simulink model "pv_control"  (R2023a)
settings: Solver=FixedStepDiscrete  StartTime=0.0  StopTime=Inf  FixedStep=Ts  RelTol=1e-3  EnableMultiTasking=on
undefined symbols (not defined in the file): dendp, denPQ, DiscIntNeverNeededParam, Down, Emax, fff, GPTRIP1SEL, GPTRIP2SEL, k, Kic, Kiv, Kpc, Kpv, L, l, m, n, numdp, numPQ, Ts, TZ1, TZ2, Up, Vdc, w
libraries: memblks x14, simulink x13, c2802xlib x12, slpidlib x9, c2837xDlib x7, spsdq0toabcLib x2, spsabctodq0Lib x2, dspswit3 x2, eeGeneralControl x1, idelinklib_common x1, spsPowerdq0InstantaneousLib x1, simulink_extras x1
(part 2 of 8)

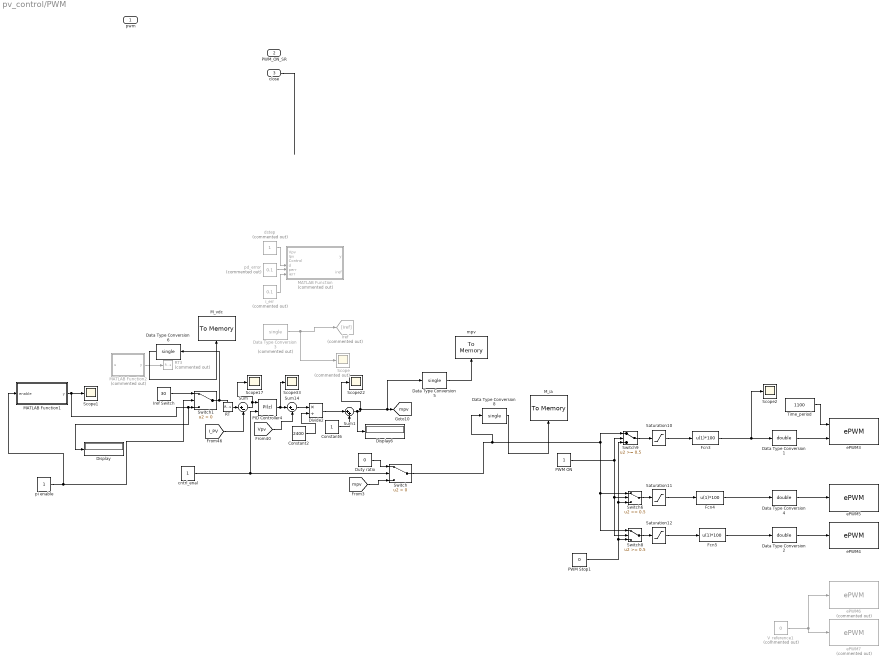
== system pv_control/PWM ==
  pwm : Inport
  PWM_ON_SR : Inport  Port=2
  close : Inport  Port=3
  Constant2 : Constant  Value=2400
  Constant6 : Constant
  Data Type Conversion1 : DataTypeConversion  OutDataTypeStr=double  SaturateOnIntegerOverflow=off  RndMeth=Floor
  Data Type Conversion2 : DataTypeConversion  OutDataTypeStr=double  SaturateOnIntegerOverflow=off  RndMeth=Floor
  Data Type Conversion3 : DataTypeConversion  Commented=on  OutDataTypeStr=single  SaturateOnIntegerOverflow=off  RndMeth=Floor
  Data Type Conversion4 : DataTypeConversion  OutDataTypeStr=double  SaturateOnIntegerOverflow=off  RndMeth=Floor
  Data Type Conversion5 : DataTypeConversion  OutDataTypeStr=single  SaturateOnIntegerOverflow=off  RndMeth=Floor
  Data Type Conversion6 : DataTypeConversion  OutDataTypeStr=single  SaturateOnIntegerOverflow=off  RndMeth=Floor
  Data Type Conversion8 : DataTypeConversion  OutDataTypeStr=single  SaturateOnIntegerOverflow=off  RndMeth=Floor
  Display : Display
  Display6 : Display
  Divide2 : Product  Inputs=*/
  Duty ratio : Constant  Value=0  OutDataTypeStr=double  SampleTime=Ts
  Fcn3 : Fcn  Expr=u(1)*100
  Fcn4 : Fcn  Expr=u(1)*100
  Fcn5 : Fcn  Expr=u(1)*100
  Iref : Goto  Commented=on  GotoTag=Iref
  Iref Switch : Constant  Value=30
  MATLAB Function : MATLAB Function  Commented=on  TreatAsAtomicUnit=on  SystemSampleTime=0.1
  MATLAB Function1 : MATLAB Function  TreatAsAtomicUnit=on  SystemSampleTime=0.0005
  MATLAB Function2 : MATLAB Function  Commented=on  TreatAsAtomicUnit=on  SystemSampleTime=0.1
  M_ia : memblks/To Memory  memAddressMask=a800  dType=single  useInitValue=off  initValue=0  useTermValue=off  termValue=0  isRealtimeEnabled=on  emitCCBeforeWrite=off  emitCCAfterWrite=on  CCAfterWrite=if(n4<200) ia[n4++]=*ia_pointer;else n4=0;
  M_vdc : memblks/To Memory  memAddressMask=a300  dType=single  useInitValue=off  initValue=0  useTermValue=off  termValue=0  isRealtimeEnabled=on  emitCCBeforeWrite=off  emitCCAfterWrite=on  CCAfterWrite=if(n7<200) vdc[n7++]=*vdc_pointer;else n7=0;
  PID Controller4 : slpidlib/PID Controller  Controller=PI  Form=Parallel  TimeDomain=Discrete-time  UseExternalTs=off  SampleTime=Ts  IntegratorMethod=Forward Euler  FilterMethod=Forward Euler  ControllerParametersSource=internal  P=1  I=40  UseKiTs=off  D=0  N=100  UseFilter=on  TunerSelectOption=Frequency Response Based  InitialConditionSource=internal  InitialConditionForIntegrator=0  InitialConditionForFilter=0  DifferentiatorICPrevScaledInput=0  ExternalReset=level  TrackingMode=off  Kt=1  LimitOutput=off  SatLimitsSource=internal  UpperSaturationLimit=inf  LowerSaturationLimit=-inf  LinearizeAsGain=on  AntiWindupMode=none  Kb=1  LimitIntegrator=off  UpperIntegratorSaturationLimit=inf  LowerIntegratorSaturationLimit=-inf  POutMin=[]  POutMax=[]  IOutMin=[]  IOutMax=[]  DOutMin=[]  DOutMax=[]  NOutMin=[]  NOutMax=[]  SumOutMin=[]  SumOutMax=[]  SaturationOutMin=[]  SaturationOutMax=[]  PParamMin=[]  PParamMax=[]  IParamMin=[]  IParamMax=[]  DParamMin=[]  DParamMax=[]  NParamMin=[]  NParamMax=[]  KbParamMin=[]  KbParamMax=[]  KtParamMin=[]  KtParamMax=[]  KbOutMin=[]  KbOutMax=[]  KtOutMin=[]  KtOutMax=[]  IntegratorOutMin=[]  IntegratorOutMax=[]  FilterOutMin=[]  FilterOutMax=[]  SumI1OutMin=[]  SumI1OutMax=[]  SumI2OutMin=[]  SumI2OutMax=[]  SumI3OutMin=[]  SumI3OutMax=[]  SumI4OutMin=[]  SumI4OutMax=[]  SumDOutMin=[]  SumDOutMax=[]  DifferentiatorOutMin=[]  DifferentiatorOutMax=[]  FilterDiffOutCoefMin=[]  FilterDiffOutCoefMax=[]  ReciprocalOutMin=[]  ReciprocalOutMax=[]  SumDenOutMin=[]  SumDenOutMax=[]  SumNumOutMin=[]  SumNumOutMax=[]  DivideOutMin=[]  DivideOutMax=[]  UdiffTsProdOutMin=[]  UdiffTsProdOutMax=[]  NTsProdOutMin=[]  NTsProdOutMax=[]  UintegralTsProdOutMin=[]  UintegralTsProdOutMax=[]  UngainTsProdOutMin=[]  UngainTsProdOutMax=[]  ClampingZeroOutDataTypeStr=Inherit: Inherit via back propagation  ClampingZeroOutMin=[]  ClampingZeroOutMax=[]  FilterDenConstantOutDataTypeStr=Inherit: Inherit via back propagation  FilterDenConstantOutMin=[]  FilterDenConstantOutMax=[]  PCopyOutDataTypeStr=Inherit: Inherit via back propagation  PCopyOutMin=[]  PCopyOutMax=[]  NCopyOutDataTypeStr=Inherit: Inherit via back propagation  NCopyOutMin=[]  NCopyOutMax=[]  IntegratorContinuousStateAttributes=''  IntegratorStateMustResolveToSignalObject=off  IntegratorRTWStateStorageClass=Auto  FilterContinuousStateAttributes=''  FilterStateMustResolveToSignalObject=off  FilterRTWStateStorageClass=Auto  ParallelPVariant=InternalParameters  IdealPVariant=Disabled  IVariant=InternalParameters  DVariant=Disabled  IntegratorVariant=Discrete  SatVariant=Disabled  AWVariant=Passthrough  PCopyVariant=Disabled  TRVariant=Disabled  FdbkBlocksVariant=Forward  IdealPFdbkVariant=Disabled  SatFdbkVariant=Disabled  DerivativeFilterVariant=Disabled  NVariant=Disabled  NCopyVariant=Disabled_SignalSpec  FilterICVariant=Disabled  IntegratorICVariant=InternalICs  ExternalResetVariant=ExternalReset  TRSumVariant=Passthrough  SumFdbkVariant=Disabled  SumVariant=Sum_PI  TsampFilterVariant=InternalTs  TsampNgainVariant=Passthrough  TsampIntegralVariant=Disabled_SignalSpec  ExternalSaturationOutDataTypeStr=Inherit: Same as second input
  PWM ON : Constant
  PWM Stop1 : Constant  Value=0  OutDataTypeStr=single  SampleTime=Ts
  RT : RateTransition  OutPortSampleTime=1e-05
  RT3 : RateTransition  Commented=on  OutPortSampleTime=Ts
  Saturation10 : Saturate  UpperLimit=1  LowerLimit=0  OutDataTypeStr=double
  Saturation11 : Saturate  UpperLimit=1  LowerLimit=0  OutDataTypeStr=double
  Saturation12 : Saturate  UpperLimit=1  LowerLimit=0  OutDataTypeStr=double
  Scope : Scope  Commented=on
  Scope{1..2,17,22,33} (5 alike) : Scope
  Sum : Sum  Inputs=|+-
  Sum1 : Sum  Inputs=|++
  Sum14 : Sum  Inputs=|+-
  Switch : Switch  Criteria=u2 > Threshold  SaturateOnIntegerOverflow=off  InputSameDT=off
  Switch1 : Switch  Criteria=u2 > Threshold  OutDataTypeStr=single  SaturateOnIntegerOverflow=off  InputSameDT=off
  Switch6 : Switch  Threshold=0.5  OutDataTypeStr=single  SaturateOnIntegerOverflow=off  InputSameDT=off
  Switch8 : Switch  Threshold=0.5  OutDataTypeStr=single  SaturateOnIntegerOverflow=off  InputSameDT=off
  Switch9 : Switch  Threshold=0.5  OutDataTypeStr=single  SaturateOnIntegerOverflow=off  InputSameDT=off
  Time_period : Constant  Value=1100  OutDataTypeStr=double  SampleTime=Ts
  V_reference1 : Constant  Commented=on  Value=0  OutDataTypeStr=double  SampleTime=Ts
  cntrl_enal : Constant
  dstep : Constant  Commented=on  OutDataTypeStr=single
  ePWM3 : c2802xlib/ePWM  PwmType=C2000_Type4  useModule=ePWM4  ePWMxLINKTBPRD=Not Linked  periodUnits=Clock cycles  timerSource=Input port  timerPeriod_clk=10000  timerPeriod_sec=0.0001  tbshadow=Counter equals to zero  countingMode=Up-Down  phaseActiveEnable=Disable  phaseDirection=Count up after sync  phaseActive=0  synchronizationEnable=off  dcaevt1Sync=off  dcbevt1Sync=off  synchronizationOption=Disable  dcbevt1SyncOut=off  dcaevt1SyncOut=off  cmpdSyncOut=off  cmpcSyncOut=off  cmpbSyncOut=off  zeroSyncOut=off  swfSyncOut=off  perSynchronizationOption=Counter equals to period (CTR=PRD)  clockPrescale=1  HSclockPrescale=1  enswap=off  ePWMxAStatus=on  ePWMxAactionLogic1=Set  ePWMxAactionLogic2=Do nothing  ePWMxAactionLogic3=Clear  ePWMxAactionLogic4=Set  ePWMxAactionLogic5=Do nothing  ePWMxAactionLogic6=Do nothing  ePWMxACSFenable=off  ePWMxACSFvalue=Forcing disable  ePWMxASFreload=Zero  ePWMxBStatus=off  ePWMxBactionLogic1=Set  ePWMxBactionLogic2=Do nothing  ePWMxBactionLogic3=Clear  ePWMxBactionLogic4=Set  ePWMxBactionLogic5=Do nothing  ePWMxBactionLogic6=Do nothing  ePWMxBCSFenable=off  ePWMxBCSFvalue=Forcing low  ePWMxBSFreload=Zero  ePWNxBOutWay=off  ePWMxLINKCMPA=Not Linked  CMPAUnits=Percentages  CMPASource=Input port  CMPAValue_per=0  CMPAValue_clk=0  enCMPAshadow=Counter equals to zero (CTR=Zero)  ePWMxLINKCMPB=Not Linked  CMPBUnits=Clock cycles  CMPBSource=Specify via dialog  CMPBValue_per=50  CMPBValue_clk=3277  enCMPBshadow=Counter equals to zero (CTR=Zero)  ePWMxLINKCMPC=Not Linked  CMPCUnits=Clock cycles  CMPCSource=Specify via dialog  CMPCValue_per=50  CMPCValue_clk=3277  enCMPCshadow=Counter equals to zero (CTR=Zero)  ePWMxLINKCMPD=Not Linked  CMPDUnits=Clock cycles  CMPDSource=Specify via dialog  CMPDValue_per=50  CMPDValue_clk=3277  enCMPDshadow=Counter equals to zero (CTR=Zero)  enableDBePWMxA=on  enableDBePWMxB=on  enhalfcycle=off  DBpolarity=Active high complementary (AHC)  DBedgeDelay=Positive  DBSource_ePWMxA=ePWMxA  DBSource_ePWMxB=ePWMxA  DBPeriodUnits=Clock cycles  DBperiodSource=Specify via dialog  REDperiod=122  FEDperiod=122  REDperiod_sec=0  FEDperiod_sec=0  LoadModeDBRED=Immediate without using shadow  LoadModeDBFED=Immediate without using shadow  adcstartModuleA=on  adcrequestEventA=First event  adcstartEventA=Digital Compare Module A Event 1 start of conversion (DCAEVT1.soc)  adcstartEventA_type2=Counter equals to zero or period (CTR=Zero or CTR=PRD)  adcstartModuleB=off  adcrequestEventB=First event  adcstartEventB=Counter equals to zero (CTR=Zero)  adcstartEventB_type2=Counter equals to zero (CTR=Zero)  intEn=off  intPrd=First event  intSel=Counter equals to zero (CTR=Zero)  intSel_type2=Counter equals to zero (CTR=Zero)  hrpe=on  enHRPWM=on  HRPWM_LoadMode=Counter equals to period (CTR=PRD)  HRPWM_CTLMode=Duty or Period control mode  HRPWM_EDGMode=Both edge  hrpeb=off  enHRPWMB=off  HRPWM_LoadModeB=Counter equals to zero (CTR=ZERO)  HRPWM_CTLModeB=Duty or Period control mode  HRPWM_EDGModeB=Both edge  enHRDBRED=off  enHRDBFED=off  enSFO=on  enautoconv=on  chopperEnable=off  chopperFrequency=1  chopperFirstwidth=1  chopperDuty=12.5%  tripZonesource=Specify via dialog  tzselOSHT1=off  tzselOSHT2=off  tzselOSHT3=off  tzselOSHDCAEV1=off  tzselOSHDCBEV1=off  tzselCBC1=off  tzselCBC2=off  tzselCBC3=off  tzselCBCDCAEV2=off  tzselCBCDCBEV2=off  tzselOSHT4=off  tzselOSHT5=off  tzselOSHT6=off  tzselCBC4=off  tzselCBC5=off  tzselCBC6=off  enTzOstIntr=off  enTzCbcIntr=off  enTzDCAEVT1Intr=off  enTzDCAEVT2Intr=off  enTzDCBEVT1Intr=off  enTzDCBEVT2Intr=off  ePWMxAforced=No action  ePWMxBforced=No action  DCAEVT1forced=No action  DCBEVT1forced=No action  DCAEVT2forced=No action  DCBEVT2forced=No action  dcah=Trip Zone 1 input (TZ1)  dcal=Trip Zone 2 input (TZ2)  dcbh=Trip Zone 1 input (TZ1)  dcbl=Trip Zone 2 input (TZ2)  dcah_type2=GPTRIP1SEL/(TZ1)  dcal_type2=GPTRIP2SEL/(TZ2)  dcbh_type2=GPTRIP1SEL/(TZ1)  dcbl_type2=GPTRIP2SEL/(TZ2)  gendcaevt1=Event disabled  gendcaevt2=Event disabled  gendcbevt1=Event disabled  gendcbevt2=Event disabled  dcaevt1src=DCAEVT1 with sync  dcaevt2src=DCAEVT2 with sync  dcbevt1src=DCBEVT1 with sync  dcbevt2src=DCBEVT2 with sync  pulsesel=Counter equals to zero (CTR=Zero)  blankinv=off  blankoffset=0  blankwidth=0  evsrcsel=Filtered version of DCAEVT1 (DCAEVT1FILT)  encape=off
  ePWM4 : c2802xlib/ePWM  PwmType=C2000_Type4  useModule=ePWM3  ePWMxLINKTBPRD=Not Linked  periodUnits=Clock cycles  timerSource=Specify via dialog  timerPeriod_clk=4687  timerPeriod_sec=0.0001  tbshadow=Counter equals to zero  countingMode=Up-Down  phaseActiveEnable=Disable  phaseDirection=Count down after sync  phaseActive=0  synchronizationEnable=off  dcaevt1Sync=off  dcbevt1Sync=off  synchronizationOption=Disable  dcbevt1SyncOut=off  dcaevt1SyncOut=off  cmpdSyncOut=off  cmpcSyncOut=off  cmpbSyncOut=off  zeroSyncOut=off  swfSyncOut=off  perSynchronizationOption=Counter equals to period (CTR=PRD)  clockPrescale=1  HSclockPrescale=1  enswap=off  ePWMxAStatus=on  ePWMxAactionLogic1=Set  ePWMxAactionLogic2=Do nothing  ePWMxAactionLogic3=Clear  ePWMxAactionLogic4=Set  ePWMxAactionLogic5=Do nothing  ePWMxAactionLogic6=Do nothing  ePWMxACSFenable=off  ePWMxACSFvalue=Forcing disable  ePWMxASFreload=Zero  ePWMxBStatus=off  ePWMxBactionLogic1=Set  ePWMxBactionLogic2=Do nothing  ePWMxBactionLogic3=Clear  ePWMxBactionLogic4=Set  ePWMxBactionLogic5=Do nothing  ePWMxBactionLogic6=Do nothing  ePWMxBCSFenable=off  ePWMxBCSFvalue=Forcing disable  ePWMxBSFreload=Zero  ePWNxBOutWay=on  ePWMxLINKCMPA=Not Linked  CMPAUnits=Percentages  CMPASource=Input port  CMPAValue_per=0  CMPAValue_clk=0  enCMPAshadow=Counter equals to zero (CTR=Zero)  ePWMxLINKCMPB=Not Linked  CMPBUnits=Clock cycles  CMPBSource=Specify via dialog  CMPBValue_per=50  CMPBValue_clk=3277  enCMPBshadow=Counter equals to zero (CTR=Zero)  ePWMxLINKCMPC=Not Linked  CMPCUnits=Clock cycles  CMPCSource=Specify via dialog  CMPCValue_per=50  CMPCValue_clk=3277  enCMPCshadow=Counter equals to zero (CTR=Zero)  ePWMxLINKCMPD=Not Linked  CMPDUnits=Clock cycles  CMPDSource=Specify via dialog  CMPDValue_per=50  CMPDValue_clk=3277  enCMPDshadow=Counter equals to zero (CTR=Zero)  enableDBePWMxA=on  enableDBePWMxB=on  enhalfcycle=off  DBpolarity=Active high complementary (AHC)  DBedgeDelay=Positive  DBSource_ePWMxA=ePWMxA  DBSource_ePWMxB=ePWMxA  DBPeriodUnits=Clock cycles  DBperiodSource=Specify via dialog  REDperiod=122  FEDperiod=122  REDperiod_sec=0  FEDperiod_sec=0  LoadModeDBRED=Immediate without using shadow  LoadModeDBFED=Immediate without using shadow  adcstartModuleA=off  adcrequestEventA=First event  adcstartEventA=Digital Compare Module A Event 1 start of conversion (DCAEVT1.soc)  adcstartEventA_type2=Counter equals to zero or period (CTR=Zero or CTR=PRD)  adcstartModuleB=off  adcrequestEventB=First event  adcstartEventB=Counter equals to zero (CTR=Zero)  adcstartEventB_type2=Counter equals to zero (CTR=Zero)  intEn=off  intPrd=First event  intSel=Counter equals to zero (CTR=Zero)  intSel_type2=Counter equals to zero (CTR=Zero)  hrpe=on  enHRPWM=on  HRPWM_LoadMode=Counter equals to period (CTR=PRD)  HRPWM_CTLMode=Duty or Period control mode  HRPWM_EDGMode=Both edge  hrpeb=off  enHRPWMB=off  HRPWM_LoadModeB=Counter equals to zero (CTR=ZERO)  HRPWM_CTLModeB=Duty or Period control mode  HRPWM_EDGModeB=Both edge  enHRDBRED=off  enHRDBFED=off  enSFO=on  enautoconv=on  chopperEnable=off  chopperFrequency=1  chopperFirstwidth=1  chopperDuty=12.5%  tripZonesource=Specify via dialog  tzselOSHT1=off  tzselOSHT2=off  tzselOSHT3=off  tzselOSHDCAEV1=off  tzselOSHDCBEV1=off  tzselCBC1=off  tzselCBC2=off  tzselCBC3=off  tzselCBCDCAEV2=off  tzselCBCDCBEV2=off  tzselOSHT4=off  tzselOSHT5=off  tzselOSHT6=off  tzselCBC4=off  tzselCBC5=off  tzselCBC6=off  enTzOstIntr=off  enTzCbcIntr=off  enTzDCAEVT1Intr=off  enTzDCAEVT2Intr=off  enTzDCBEVT1Intr=off  enTzDCBEVT2Intr=off  ePWMxAforced=No action  ePWMxBforced=No action  DCAEVT1forced=No action  DCBEVT1forced=No action  DCAEVT2forced=No action  DCBEVT2forced=No action  dcah=Trip Zone 1 input (TZ1)  dcal=Trip Zone 2 input (TZ2)  dcbh=Trip Zone 1 input (TZ1)  dcbl=Trip Zone 2 input (TZ2)  dcah_type2=GPTRIP1SEL/(TZ1)  dcal_type2=GPTRIP2SEL/(TZ2)  dcbh_type2=GPTRIP1SEL/(TZ1)  dcbl_type2=GPTRIP2SEL/(TZ2)  gendcaevt1=Event disabled  gendcaevt2=Event disabled  gendcbevt1=Event disabled  gendcbevt2=Event disabled  dcaevt1src=DCAEVT1 with sync  dcaevt2src=DCAEVT2 with sync  dcbevt1src=DCBEVT1 with sync  dcbevt2src=DCBEVT2 with sync  pulsesel=Counter equals to zero (CTR=Zero)  blankinv=off  blankoffset=0  blankwidth=0  evsrcsel=Filtered version of DCAEVT1 (DCAEVT1FILT)  encape=off
  ePWM5 : c2802xlib/ePWM  PwmType=C2000_Type4  useModule=ePWM2  ePWMxLINKTBPRD=Not Linked  periodUnits=Clock cycles  timerSource=Specify via dialog  timerPeriod_clk=4687  timerPeriod_sec=0.0001  tbshadow=Counter equals to zero  countingMode=Up-Down  phaseActiveEnable=Disable  phaseDirection=Count down after sync  phaseActive=0  synchronizationEnable=off  dcaevt1Sync=off  dcbevt1Sync=off  synchronizationOption=Disable  dcbevt1SyncOut=off  dcaevt1SyncOut=off  cmpdSyncOut=off  cmpcSyncOut=off  cmpbSyncOut=off  zeroSyncOut=off  swfSyncOut=off  perSynchronizationOption=Counter equals to period (CTR=PRD)  clockPrescale=1  HSclockPrescale=1  enswap=off  ePWMxAStatus=on  ePWMxAactionLogic1=Set  ePWMxAactionLogic2=Do nothing  ePWMxAactionLogic3=Clear  ePWMxAactionLogic4=Set  ePWMxAactionLogic5=Do nothing  ePWMxAactionLogic6=Do nothing  ePWMxACSFenable=off  ePWMxACSFvalue=Forcing disable  ePWMxASFreload=Zero  ePWMxBStatus=on  ePWMxBactionLogic1=Set  ePWMxBactionLogic2=Do nothing  ePWMxBactionLogic3=Clear  ePWMxBactionLogic4=Set  ePWMxBactionLogic5=Do nothing  ePWMxBactionLogic6=Do nothing  ePWMxBCSFenable=off  ePWMxBCSFvalue=Forcing disable  ePWMxBSFreload=Zero  ePWNxBOutWay=on  ePWMxLINKCMPA=Not Linked  CMPAUnits=Percentages  CMPASource=Input port  CMPAValue_per=0  CMPAValue_clk=0  enCMPAshadow=Counter equals to zero (CTR=Zero)  ePWMxLINKCMPB=Not Linked  CMPBUnits=Clock cycles  CMPBSource=Specify via dialog  CMPBValue_per=50  CMPBValue_clk=3277  enCMPBshadow=Counter equals to zero (CTR=Zero)  ePWMxLINKCMPC=Not Linked  CMPCUnits=Clock cycles  CMPCSource=Specify via dialog  CMPCValue_per=50  CMPCValue_clk=3277  enCMPCshadow=Counter equals to zero (CTR=Zero)  ePWMxLINKCMPD=Not Linked  CMPDUnits=Clock cycles  CMPDSource=Specify via dialog  CMPDValue_per=50  CMPDValue_clk=3277  enCMPDshadow=Counter equals to zero (CTR=Zero)  enableDBePWMxA=on  enableDBePWMxB=on  enhalfcycle=off  DBpolarity=Active high complementary (AHC)  DBedgeDelay=Positive  DBSource_ePWMxA=ePWMxA  DBSource_ePWMxB=ePWMxA  DBPeriodUnits=Clock cycles  DBperiodSource=Specify via dialog  REDperiod=122  FEDperiod=122  REDperiod_sec=0  FEDperiod_sec=0  LoadModeDBRED=Immediate without using shadow  LoadModeDBFED=Immediate without using shadow  adcstartModuleA=on  adcrequestEventA=First event  adcstartEventA=Digital Compare Module A Event 1 start of conversion (DCAEVT1.soc)  adcstartEventA_type2=Counter equals to zero or period (CTR=Zero or CTR=PRD)  adcstartModuleB=off  adcrequestEventB=First event  adcstartEventB=Counter equals to zero (CTR=Zero)  adcstartEventB_type2=Counter equals to zero (CTR=Zero)  intEn=off  intPrd=First event  intSel=Counter equals to zero (CTR=Zero)  intSel_type2=Counter equals to zero (CTR=Zero)  hrpe=on  enHRPWM=on  HRPWM_LoadMode=Counter equals to period (CTR=PRD)  HRPWM_CTLMode=Duty or Period control mode  HRPWM_EDGMode=Both edge  hrpeb=off  enHRPWMB=off  HRPWM_LoadModeB=Counter equals to zero (CTR=ZERO)  HRPWM_CTLModeB=Duty or Period control mode  HRPWM_EDGModeB=Both edge  enHRDBRED=off  enHRDBFED=off  enSFO=on  enautoconv=on  chopperEnable=off  chopperFrequency=1  chopperFirstwidth=1  chopperDuty=12.5%  tripZonesource=Specify via dialog  tzselOSHT1=off  tzselOSHT2=off  tzselOSHT3=off  tzselOSHDCAEV1=off  tzselOSHDCBEV1=off  tzselCBC1=off  tzselCBC2=off  tzselCBC3=off  tzselCBCDCAEV2=off  tzselCBCDCBEV2=off  tzselOSHT4=off  tzselOSHT5=off  tzselOSHT6=off  tzselCBC4=off  tzselCBC5=off  tzselCBC6=off  enTzOstIntr=off  enTzCbcIntr=off  enTzDCAEVT1Intr=off  enTzDCAEVT2Intr=off  enTzDCBEVT1Intr=off  enTzDCBEVT2Intr=off  ePWMxAforced=No action  ePWMxBforced=No action  DCAEVT1forced=No action  DCBEVT1forced=No action  DCAEVT2forced=No action  DCBEVT2forced=No action  dcah=Trip Zone 1 input (TZ1)  dcal=Trip Zone 2 input (TZ2)  dcbh=Trip Zone 1 input (TZ1)  dcbl=Trip Zone 2 input (TZ2)  dcah_type2=GPTRIP1SEL/(TZ1)  dcal_type2=GPTRIP2SEL/(TZ2)  dcbh_type2=GPTRIP1SEL/(TZ1)  dcbl_type2=GPTRIP2SEL/(TZ2)  gendcaevt1=Event disabled  gendcaevt2=Event disabled  gendcbevt1=Event disabled  gendcbevt2=Event disabled  dcaevt1src=DCAEVT1 with sync  dcaevt2src=DCAEVT2 with sync  dcbevt1src=DCBEVT1 with sync  dcbevt2src=DCBEVT2 with sync  pulsesel=Counter equals to zero (CTR=Zero)  blankinv=off  blankoffset=0  blankwidth=0  evsrcsel=Filtered version of DCAEVT1 (DCAEVT1FILT)  encape=off
  ePWM6 : c2802xlib/ePWM  Commented=on  PwmType=C2000_Type4  useModule=ePWM5  ePWMxLINKTBPRD=Not Linked  periodUnits=Clock cycles  timerSource=Specify via dialog  timerPeriod_clk=4687  timerPeriod_sec=0.0001  tbshadow=Counter equals to zero  countingMode=Up-Down  phaseActiveEnable=Disable  phaseDirection=Count down after sync  phaseActive=0  synchronizationEnable=off  dcaevt1Sync=off  dcbevt1Sync=off  synchronizationOption=Disable  dcbevt1SyncOut=off  dcaevt1SyncOut=off  cmpdSyncOut=off  cmpcSyncOut=off  cmpbSyncOut=off  zeroSyncOut=off  swfSyncOut=off  perSynchronizationOption=Counter equals to period (CTR=PRD)  clockPrescale=1  HSclockPrescale=1  enswap=off  ePWMxAStatus=on  ePWMxAactionLogic1=Set  ePWMxAactionLogic2=Do nothing  ePWMxAactionLogic3=Clear  ePWMxAactionLogic4=Set  ePWMxAactionLogic5=Do nothing  ePWMxAactionLogic6=Do nothing  ePWMxACSFenable=off  ePWMxACSFvalue=Forcing disable  ePWMxASFreload=Zero  ePWMxBStatus=off  ePWMxBactionLogic1=Set  ePWMxBactionLogic2=Do nothing  ePWMxBactionLogic3=Clear  ePWMxBactionLogic4=Set  ePWMxBactionLogic5=Do nothing  ePWMxBactionLogic6=Do nothing  ePWMxBCSFenable=off  ePWMxBCSFvalue=Forcing disable  ePWMxBSFreload=Zero  ePWNxBOutWay=off  ePWMxLINKCMPA=Not Linked  CMPAUnits=Percentages  CMPASource=Input port  CMPAValue_per=0  CMPAValue_clk=0  enCMPAshadow=Counter equals to zero (CTR=Zero)  ePWMxLINKCMPB=Not Linked  CMPBUnits=Clock cycles  CMPBSource=Specify via dialog  CMPBValue_per=50  CMPBValue_clk=3277  enCMPBshadow=Counter equals to zero (CTR=Zero)  ePWMxLINKCMPC=Not Linked  CMPCUnits=Clock cycles  CMPCSource=Specify via dialog  CMPCValue_per=50  CMPCValue_clk=3277  enCMPCshadow=Counter equals to zero (CTR=Zero)  ePWMxLINKCMPD=Not Linked  CMPDUnits=Clock cycles  CMPDSource=Specify via dialog  CMPDValue_per=50  CMPDValue_clk=3277  enCMPDshadow=Counter equals to zero (CTR=Zero)  enableDBePWMxA=on  enableDBePWMxB=on  enhalfcycle=off  DBpolarity=Active high complementary (AHC)  DBedgeDelay=Positive  DBSource_ePWMxA=ePWMxA  DBSource_ePWMxB=ePWMxA  DBPeriodUnits=Clock cycles  DBperiodSource=Specify via dialog  REDperiod=122  FEDperiod=122  REDperiod_sec=0  FEDperiod_sec=0  LoadModeDBRED=Immediate without using shadow  LoadModeDBFED=Immediate without using shadow  adcstartModuleA=on  adcrequestEventA=First event  adcstartEventA=Digital Compare Module A Event 1 start of conversion (DCAEVT1.soc)  adcstartEventA_type2=Counter equals to zero or period (CTR=Zero or CTR=PRD)  adcstartModuleB=off  adcrequestEventB=First event  adcstartEventB=Counter equals to zero (CTR=Zero)  adcstartEventB_type2=Counter equals to zero (CTR=Zero)  intEn=off  intPrd=First event  intSel=Counter equals to zero (CTR=Zero)  intSel_type2=Counter equals to zero (CTR=Zero)  hrpe=on  enHRPWM=on  HRPWM_LoadMode=Counter equals to period (CTR=PRD)  HRPWM_CTLMode=Duty or Period control mode  HRPWM_EDGMode=Both edge  hrpeb=off  enHRPWMB=off  HRPWM_LoadModeB=Counter equals to zero (CTR=ZERO)  HRPWM_CTLModeB=Duty or Period control mode  HRPWM_EDGModeB=Both edge  enHRDBRED=off  enHRDBFED=off  enSFO=on  enautoconv=on  chopperEnable=off  chopperFrequency=1  chopperFirstwidth=1  chopperDuty=12.5%  tripZonesource=Specify via dialog  tzselOSHT1=off  tzselOSHT2=off  tzselOSHT3=off  tzselOSHDCAEV1=off  tzselOSHDCBEV1=off  tzselCBC1=off  tzselCBC2=off  tzselCBC3=off  tzselCBCDCAEV2=off  tzselCBCDCBEV2=off  tzselOSHT4=off  tzselOSHT5=off  tzselOSHT6=off  tzselCBC4=off  tzselCBC5=off  tzselCBC6=off  enTzOstIntr=off  enTzCbcIntr=off  enTzDCAEVT1Intr=off  enTzDCAEVT2Intr=off  enTzDCBEVT1Intr=off  enTzDCBEVT2Intr=off  ePWMxAforced=No action  ePWMxBforced=No action  DCAEVT1forced=No action  DCBEVT1forced=No action  DCAEVT2forced=No action  DCBEVT2forced=No action  dcah=Trip Zone 1 input (TZ1)  dcal=Trip Zone 2 input (TZ2)  dcbh=Trip Zone 1 input (TZ1)  dcbl=Trip Zone 2 input (TZ2)  dcah_type2=GPTRIP1SEL/(TZ1)  dcal_type2=GPTRIP2SEL/(TZ2)  dcbh_type2=GPTRIP1SEL/(TZ1)  dcbl_type2=GPTRIP2SEL/(TZ2)  gendcaevt1=Event disabled  gendcaevt2=Event disabled  gendcbevt1=Event disabled  gendcbevt2=Event disabled  dcaevt1src=DCAEVT1 with sync  dcaevt2src=DCAEVT2 with sync  dcbevt1src=DCBEVT1 with sync  dcbevt2src=DCBEVT2 with sync  pulsesel=Counter equals to zero (CTR=Zero)  blankinv=off  blankoffset=0  blankwidth=0  evsrcsel=Filtered version of DCAEVT1 (DCAEVT1FILT)  encape=off
  ePWM7 : c2802xlib/ePWM  Commented=on  PwmType=C2000_Type4  useModule=ePWM6  ePWMxLINKTBPRD=Not Linked  periodUnits=Clock cycles  timerSource=Specify via dialog  timerPeriod_clk=4687  timerPeriod_sec=0.0001  tbshadow=Counter equals to zero  countingMode=Up-Down  phaseActiveEnable=Disable  phaseDirection=Count down after sync  phaseActive=0  synchronizationEnable=off  dcaevt1Sync=off  dcbevt1Sync=off  synchronizationOption=Disable  dcbevt1SyncOut=off  dcaevt1SyncOut=off  cmpdSyncOut=off  cmpcSyncOut=off  cmpbSyncOut=off  zeroSyncOut=off  swfSyncOut=off  perSynchronizationOption=Counter equals to period (CTR=PRD)  clockPrescale=1  HSclockPrescale=1  enswap=off  ePWMxAStatus=on  ePWMxAactionLogic1=Set  ePWMxAactionLogic2=Do nothing  ePWMxAactionLogic3=Clear  ePWMxAactionLogic4=Set  ePWMxAactionLogic5=Do nothing  ePWMxAactionLogic6=Do nothing  ePWMxACSFenable=off  ePWMxACSFvalue=Forcing disable  ePWMxASFreload=Zero  ePWMxBStatus=off  ePWMxBactionLogic1=Set  ePWMxBactionLogic2=Do nothing  ePWMxBactionLogic3=Clear  ePWMxBactionLogic4=Set  ePWMxBactionLogic5=Do nothing  ePWMxBactionLogic6=Do nothing  ePWMxBCSFenable=off  ePWMxBCSFvalue=Forcing disable  ePWMxBSFreload=Zero  ePWNxBOutWay=off  ePWMxLINKCMPA=Not Linked  CMPAUnits=Percentages  CMPASource=Input port  CMPAValue_per=0  CMPAValue_clk=0  enCMPAshadow=Counter equals to zero (CTR=Zero)  ePWMxLINKCMPB=Not Linked  CMPBUnits=Clock cycles  CMPBSource=Specify via dialog  CMPBValue_per=50  CMPBValue_clk=3277  enCMPBshadow=Counter equals to zero (CTR=Zero)  ePWMxLINKCMPC=Not Linked  CMPCUnits=Clock cycles  CMPCSource=Specify via dialog  CMPCValue_per=50  CMPCValue_clk=3277  enCMPCshadow=Counter equals to zero (CTR=Zero)  ePWMxLINKCMPD=Not Linked  CMPDUnits=Clock cycles  CMPDSource=Specify via dialog  CMPDValue_per=50  CMPDValue_clk=3277  enCMPDshadow=Counter equals to zero (CTR=Zero)  enableDBePWMxA=on  enableDBePWMxB=on  enhalfcycle=off  DBpolarity=Active high complementary (AHC)  DBedgeDelay=Positive  DBSource_ePWMxA=ePWMxA  DBSource_ePWMxB=ePWMxA  DBPeriodUnits=Clock cycles  DBperiodSource=Specify via dialog  REDperiod=122  FEDperiod=122  REDperiod_sec=0  FEDperiod_sec=0  LoadModeDBRED=Immediate without using shadow  LoadModeDBFED=Immediate without using shadow  adcstartModuleA=on  adcrequestEventA=First event  adcstartEventA=Digital Compare Module A Event 1 start of conversion (DCAEVT1.soc)  adcstartEventA_type2=Counter equals to zero or period (CTR=Zero or CTR=PRD)  adcstartModuleB=off  adcrequestEventB=First event  adcstartEventB=Counter equals to zero (CTR=Zero)  adcstartEventB_type2=Counter equals to zero (CTR=Zero)  intEn=off  intPrd=First event  intSel=Counter equals to zero (CTR=Zero)  intSel_type2=Counter equals to zero (CTR=Zero)  hrpe=on  enHRPWM=on  HRPWM_LoadMode=Counter equals to period (CTR=PRD)  HRPWM_CTLMode=Duty or Period control mode  HRPWM_EDGMode=Both edge  hrpeb=off  enHRPWMB=off  HRPWM_LoadModeB=Counter equals to zero (CTR=ZERO)  HRPWM_CTLModeB=Duty or Period control mode  HRPWM_EDGModeB=Both edge  enHRDBRED=off  enHRDBFED=off  enSFO=on  enautoconv=on  chopperEnable=off  chopperFrequency=1  chopperFirstwidth=1  chopperDuty=12.5%  tripZonesource=Specify via dialog  tzselOSHT1=off  tzselOSHT2=off  tzselOSHT3=off  tzselOSHDCAEV1=off  tzselOSHDCBEV1=off  tzselCBC1=off  tzselCBC2=off  tzselCBC3=off  tzselCBCDCAEV2=off  tzselCBCDCBEV2=off  tzselOSHT4=off  tzselOSHT5=off  tzselOSHT6=off  tzselCBC4=off  tzselCBC5=off  tzselCBC6=off  enTzOstIntr=off  enTzCbcIntr=off  enTzDCAEVT1Intr=off  enTzDCAEVT2Intr=off  enTzDCBEVT1Intr=off  enTzDCBEVT2Intr=off  ePWMxAforced=No action  ePWMxBforced=No action  DCAEVT1forced=No action  DCBEVT1forced=No action  DCAEVT2forced=No action  DCBEVT2forced=No action  dcah=Trip Zone 1 input (TZ1)  dcal=Trip Zone 2 input (TZ2)  dcbh=Trip Zone 1 input (TZ1)  dcbl=Trip Zone 2 input (TZ2)  dcah_type2=GPTRIP1SEL/(TZ1)  dcal_type2=GPTRIP2SEL/(TZ2)  dcbh_type2=GPTRIP1SEL/(TZ1)  dcbl_type2=GPTRIP2SEL/(TZ2)  gendcaevt1=Event disabled  gendcaevt2=Event disabled  gendcbevt1=Event disabled  gendcbevt2=Event disabled  dcaevt1src=DCAEVT1 with sync  dcaevt2src=DCAEVT2 with sync  dcbevt1src=DCBEVT1 with sync  dcbevt2src=DCBEVT2 with sync  pulsesel=Counter equals to zero (CTR=Zero)  blankinv=off  blankoffset=0  blankwidth=0  evsrcsel=Filtered version of DCAEVT1 (DCAEVT1FILT)  encape=off
  i_err : Constant  Commented=on  Value=0.1  OutDataTypeStr=single
  mpv : memblks/To Memory  memAddressMask=a400  dType=single  useInitValue=off  initValue=0  useTermValue=off  termValue=0  isRealtimeEnabled=on  emitCCBeforeWrite=off  emitCCAfterWrite=on  CCAfterWrite=if(n13<200) test[n13++]=*test_pointer;else n13=0;
  pd_error : Constant  Commented=on  Value=0.1  OutDataTypeStr=single
  pi enable : Constant
  tag scope: mpv=global
  wires:
  close/1 -> ?
  Fcn5/1 -> Data Type Conversion2/1
  PWM ON/1 -> Switch8/2, Switch6/2, Switch9/2
  Saturation11/1 -> Fcn4/1
  Saturation10/1 -> Fcn3/1
  Switch9/1 -> Saturation10/1
  Switch8/1 -> Saturation12/1
  Switch6/1 -> Saturation11/1
  Fcn4/1 -> Data Type Conversion4/1
  PWM Stop1/1 -> Switch9/3, Switch6/3, Switch8/3
  Data Type Conversion4/1 -> ePWM5/1
  Saturation12/1 -> Fcn5/1
  Data Type Conversion2/1 -> ePWM4/1
  Switch/1 -> Data Type Conversion8/1, Switch8/1, Switch6/1, Switch9/1
  Time_period/1 -> ePWM3/1
  V_reference1/1 -> ePWM7/1, ePWM6/1
  Data Type Conversion1/1 -> ePWM3/2
  Fcn3/1 -> Scope2/1, Data Type Conversion1/1
  cntrl_enal/1 -> PID Controller4/2, Switch/2
  Constant6/1 -> Sum1/2
  PID Controller4/1 -> Scope33/1, Sum14/1
  [Vpv] -> Sum14/2
  Divide2/1 -> Sum1/1
  Sum/1 -> Scope17/1, PID Controller4/1
  [I_PV] -> Sum/2
  Sum14/1 -> Divide2/1
  [mpv] -> Switch/3
  Constant2/1 -> Divide2/2
  Duty ratio/1 -> Switch/1
  Data Type Conversion8/1 -> M_ia/1
  Data Type Conversion3/1 -> Scope/1, Iref/1
  dstep/1 -> MATLAB Function/4(d)
  pd_error/1 -> MATLAB Function/5(perr)
  i_err/1 -> MATLAB Function/6(ierr)
  Switch1/1 -> Data Type Conversion6/1, RT/1
  MATLAB Function2/1(y) -> RT3/1
  Iref Switch/1 -> Switch1/1
  Sum1/1 -> Scope22/1, Data Type Conversion5/1, [mpv], Display6/1
  Data Type Conversion5/1 -> mpv/1
  pi enable/1 -> Switch1/2, MATLAB Function1/1(enable)
  MATLAB Function1/1(y) -> Display/1, Switch1/3, Scope1/1
  Data Type Conversion6/1 -> M_vdc/1
  RT/1 -> Sum/1

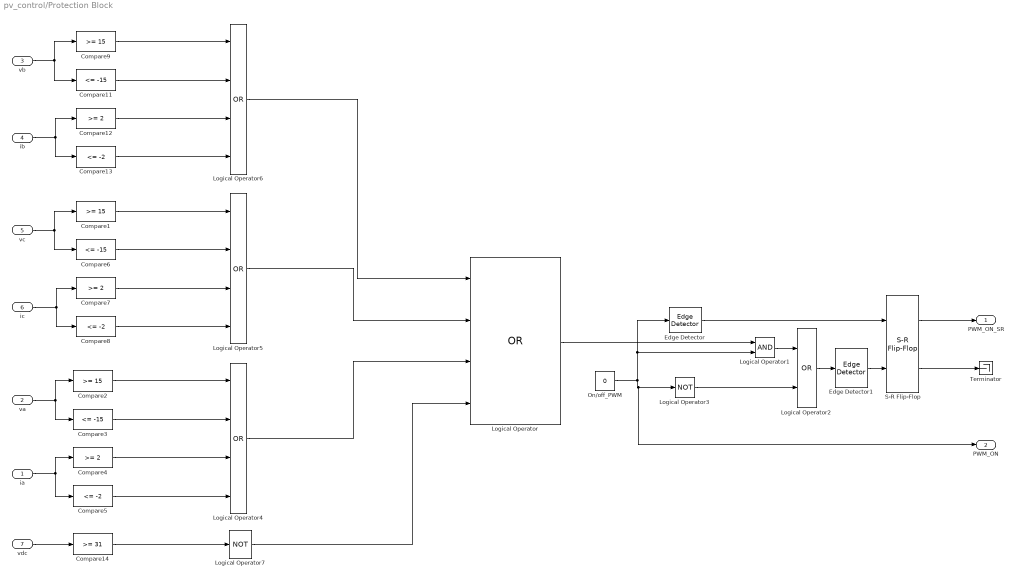
== system pv_control/Protection Block ==
  ia : Inport
  va : Inport  Port=2
  vb : Inport  Port=3
  ib : Inport  Port=4
  vc : Inport  Port=5
  ic : Inport  Port=6
  vdc : Inport  Port=7
  Compare1 : simulink/Logic and Bit Operations/Compare To Constant  relop=>=  const=15  OutDataTypeStr=boolean  ZeroCross=off
  Compare11 : simulink/Logic and Bit Operations/Compare To Constant  relop=<=  const=-15  OutDataTypeStr=boolean  ZeroCross=off
  Compare12 : simulink/Logic and Bit Operations/Compare To Constant  relop=>=  const=2  OutDataTypeStr=boolean  ZeroCross=off
  Compare13 : simulink/Logic and Bit Operations/Compare To Constant  relop=<=  const=-2  OutDataTypeStr=boolean  ZeroCross=off
  Compare14 : simulink/Logic and Bit Operations/Compare To Constant  relop=>=  const=31  OutDataTypeStr=boolean  ZeroCross=off
  Compare2 : simulink/Logic and Bit Operations/Compare To Constant  relop=>=  const=15  OutDataTypeStr=boolean  ZeroCross=off
  Compare3 : simulink/Logic and Bit Operations/Compare To Constant  relop=<=  const=-15  OutDataTypeStr=boolean  ZeroCross=off
  Compare4 : simulink/Logic and Bit Operations/Compare To Constant  relop=>=  const=2  OutDataTypeStr=boolean  ZeroCross=off
  Compare5 : simulink/Logic and Bit Operations/Compare To Constant  relop=<=  const=-2  OutDataTypeStr=boolean  ZeroCross=off
  Compare6 : simulink/Logic and Bit Operations/Compare To Constant  relop=<=  const=-15  OutDataTypeStr=boolean  ZeroCross=off
  Compare7 : simulink/Logic and Bit Operations/Compare To Constant  relop=>=  const=2  OutDataTypeStr=boolean  ZeroCross=off
  Compare8 : simulink/Logic and Bit Operations/Compare To Constant  relop=<=  const=-2  OutDataTypeStr=boolean  ZeroCross=off
  Compare9 : simulink/Logic and Bit Operations/Compare To Constant  relop=>=  const=15  OutDataTypeStr=boolean  ZeroCross=off
  Edge Detector : dspswit3/Edge Detector  InputProcessing=Columns as channels (frame based)
  Edge Detector1 : dspswit3/Edge Detector  InputProcessing=Columns as channels (frame based)
  Logical Operator{,4..6} (4 alike) : Logic  Operator=OR  Inputs=4  AllPortsSameDT=off  OutDataTypeStr=boolean
  Logical Operator1 : Logic  AllPortsSameDT=off  OutDataTypeStr=boolean
  Logical Operator2 : Logic  Operator=OR  AllPortsSameDT=off  OutDataTypeStr=boolean
  Logical Operator3 : Logic  Operator=NOT  AllPortsSameDT=off  OutDataTypeStr=boolean
  Logical Operator7 : Logic  Operator=NOT  Inputs=1  IconShape=distinctive  AllPortsSameDT=off  OutDataTypeStr=boolean
  On/off_PWM : Constant  Value=0  OutDataTypeStr=Inherit: Inherit via back propagation  SampleTime=Ts
  S-R Flip-Flop : simulink_extras/Flip Flops/S-R Flip-Flop  initial_condition=0
  Terminator : Terminator
  PWM_ON_SR : Outport
  PWM_ON : Outport  Port=2
  wires:
  Edge Detector/1 -> S-R Flip-Flop/1
  Logical Operator1/1 -> Logical Operator2/1
  Logical Operator3/1 -> Logical Operator2/2
  On/off_PWM/1 -> PWM_ON/1, Logical Operator3/1, Edge Detector/1, Logical Operator1/2
  Edge Detector1/1 -> S-R Flip-Flop/2
  va/1 -> Compare3/1, Compare2/1
  Compare2/1 -> Logical Operator4/1
  Compare3/1 -> Logical Operator4/2
  Compare4/1 -> Logical Operator4/3
  Logical Operator/1 -> Logical Operator1/1
  ia/1 -> Compare5/1, Compare4/1
  S-R Flip-Flop/2 -> Terminator/1
  S-R Flip-Flop/1 -> PWM_ON_SR/1
  Logical Operator2/1 -> Edge Detector1/1
  Compare6/1 -> Logical Operator5/2
  Compare8/1 -> Logical Operator5/4
  Compare1/1 -> Logical Operator5/1
  Compare7/1 -> Logical Operator5/3
  Compare11/1 -> Logical Operator6/2
  Compare13/1 -> Logical Operator6/4
  Compare9/1 -> Logical Operator6/1
  Compare12/1 -> Logical Operator6/3
  Logical Operator5/1 -> Logical Operator/2
  Logical Operator6/1 -> Logical Operator/1
  vb/1 -> Compare9/1, Compare11/1
  ib/1 -> Compare13/1, Compare12/1
  vc/1 -> Compare1/1, Compare6/1
  ic/1 -> Compare7/1, Compare8/1
  vdc/1 -> Compare14/1
  Logical Operator4/1 -> Logical Operator/3
  Compare5/1 -> Logical Operator4/4
  Compare14/1 -> Logical Operator7/1
  Logical Operator7/1 -> Logical Operator/4

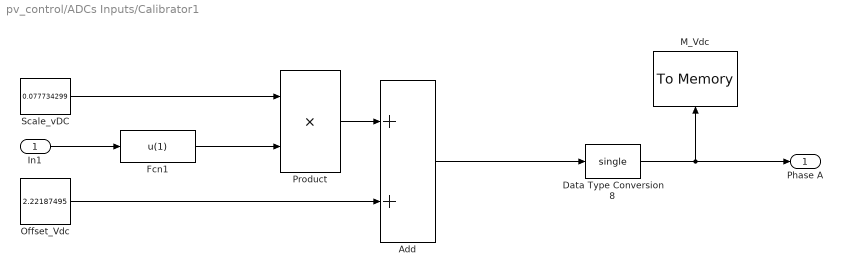
== system pv_control/ADCs Inputs/Calibrator1 ==
  In1 : Inport
  Add : Sum
  Data Type Conversion8 : DataTypeConversion  OutDataTypeStr=single  SaturateOnIntegerOverflow=off  RndMeth=Floor
  Fcn1 : Fcn  Expr=u(1)
  M_Vdc : memblks/To Memory  memAddressMask=a000  dType=single  useInitValue=off  initValue=0  useTermValue=off  termValue=0  isRealtimeEnabled=on  emitCCBeforeWrite=off  emitCCAfterWrite=on  CCAfterWrite=if(n1<200) Vdc[n1++]=*Vdc_pointer;else n1=0;
  Offset_Vdc : Constant  Value=2.22187495
  Product : Product
  Scale_vDC : Constant  Value=0.077734299
  Phase A : Outport
  wires:
  Data Type Conversion8/1 -> Phase A/1, M_Vdc/1
  Product/1 -> Add/1
  Scale_vDC/1 -> Product/1
  Fcn1/1 -> Product/2
  Offset_Vdc/1 -> Add/2
  Add/1 -> Data Type Conversion8/1
  In1/1 -> Fcn1/1

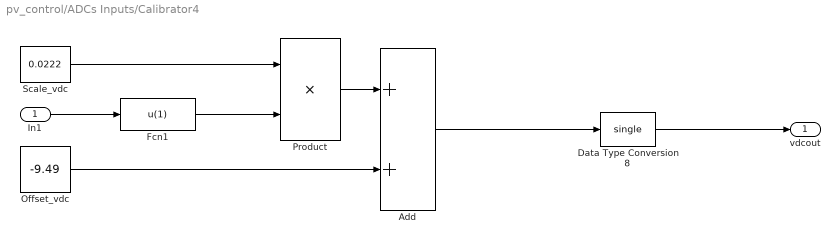
== system pv_control/ADCs Inputs/Calibrator4 ==
  In1 : Inport
  Add : Sum
  Data Type Conversion8 : DataTypeConversion  OutDataTypeStr=single  SaturateOnIntegerOverflow=off  RndMeth=Floor
  Fcn1 : Fcn  Expr=u(1)
  Offset_vdc : Constant  Value=-9.49
  Product : Product
  Scale_vdc : Constant  Value=0.0222
  "vdcout " : Outport
  wires:
  Data Type Conversion8/1 -> "vdcout "/1
  Product/1 -> Add/1
  Scale_vdc/1 -> Product/1
  Fcn1/1 -> Product/2
  Offset_vdc/1 -> Add/2
  Add/1 -> Data Type Conversion8/1
  In1/1 -> Fcn1/1

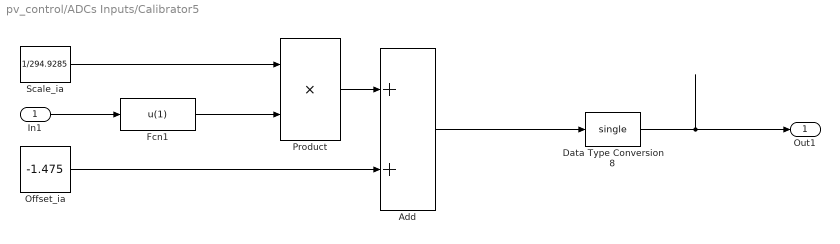
== system pv_control/ADCs Inputs/Calibrator5 ==
  In1 : Inport
  Add : Sum
  Data Type Conversion8 : DataTypeConversion  OutDataTypeStr=single  SaturateOnIntegerOverflow=off  RndMeth=Floor
  Fcn1 : Fcn  Expr=u(1)
  Offset_ia : Constant  Value=-1.475
  Product : Product
  Scale_ia : Constant  Value=1/294.9285
  Out1 : Outport
  wires:
  In1/1 -> Fcn1/1
  Add/1 -> Data Type Conversion8/1
  Offset_ia/1 -> Add/2
  Fcn1/1 -> Product/2
  Scale_ia/1 -> Product/1
  Product/1 -> Add/1
  Data Type Conversion8/1 -> Out1/1

== system pv_control/ADCs Inputs/Calibrator6 ==
  In1 : Inport
  Add : Sum
  Data Type Conversion8 : DataTypeConversion  OutDataTypeStr=single  SaturateOnIntegerOverflow=off  RndMeth=Floor
  Fcn1 : Fcn  Expr=u(1)
  Offset_ib : Constant  Value=-11.4800007
  Product : Product
  Scale_ib : Constant  Value=0.0045399997
  Iabc : Outport
  wires:
  Data Type Conversion8/1 -> Iabc/1
  Product/1 -> Add/1
  Scale_ib/1 -> Product/1
  Fcn1/1 -> Product/2
  Offset_ib/1 -> Add/2
  Add/1 -> Data Type Conversion8/1
  In1/1 -> Fcn1/1

== system pv_control/ADCs Inputs/Calibrator7 ==
  In1 : Inport
  Add : Sum
  Data Type Conversion8 : DataTypeConversion  OutDataTypeStr=single  SaturateOnIntegerOverflow=off  RndMeth=Floor
  Fcn1 : Fcn  Expr=u(1)
  Offset_ic : Constant  Value=-1.4
  Product : Product
  Scale_ic : Constant  Value=1/294.2857
  Out1 : Outport
  wires:
  In1/1 -> Fcn1/1
  Add/1 -> Data Type Conversion8/1
  Offset_ic/1 -> Add/2
  Fcn1/1 -> Product/2
  Scale_ic/1 -> Product/1
  Product/1 -> Add/1
  Data Type Conversion8/1 -> Out1/1

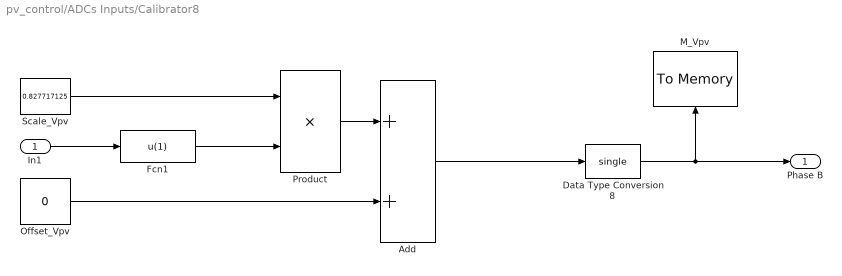
== system pv_control/ADCs Inputs/Calibrator8 ==
  In1 : Inport
  Add : Sum
  Data Type Conversion8 : DataTypeConversion  OutDataTypeStr=single  SaturateOnIntegerOverflow=off  RndMeth=Floor
  Fcn1 : Fcn  Expr=u(1)
  M_Vpv : memblks/To Memory  memAddressMask=a100  dType=single  useInitValue=off  initValue=0  useTermValue=off  termValue=0  isRealtimeEnabled=on  emitCCBeforeWrite=off  emitCCAfterWrite=on  CCAfterWrite=if(n2<200) Vpv[n2++]=*Vpv_pointer;else n2=0;
  Offset_Vpv : Constant  Value=0
  Product : Product
  Scale_Vpv : Constant  Value=0.827717125
  Phase B : Outport
  wires:
  Data Type Conversion8/1 -> Phase B/1, M_Vpv/1
  Product/1 -> Add/1
  Scale_Vpv/1 -> Product/1
  Fcn1/1 -> Product/2
  Offset_Vpv/1 -> Add/2
  Add/1 -> Data Type Conversion8/1
  In1/1 -> Fcn1/1

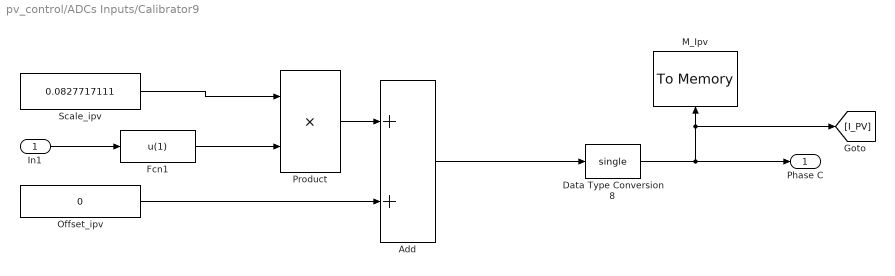
== system pv_control/ADCs Inputs/Calibrator9 ==
  In1 : Inport
  Add : Sum
  Data Type Conversion8 : DataTypeConversion  OutDataTypeStr=single  SaturateOnIntegerOverflow=off  RndMeth=Floor
  Fcn1 : Fcn  Expr=u(1)
  M_Ipv : memblks/To Memory  memAddressMask=a200  dType=single  useInitValue=off  initValue=0  useTermValue=off  termValue=0  isRealtimeEnabled=on  emitCCBeforeWrite=off  emitCCAfterWrite=on  CCAfterWrite=if(n3<200) Ipv[n3++]=*Ipv_pointer;else n3=0;
  Offset_ipv : Constant  Value=0
  Product : Product
  Scale_ipv : Constant  Value=0.0827717111
  Phase C : Outport
  wires:
  In1/1 -> Fcn1/1
  Add/1 -> Data Type Conversion8/1
  Offset_ipv/1 -> Add/2
  Fcn1/1 -> Product/2
  Scale_ipv/1 -> Product/1
  Product/1 -> Add/1
  Data Type Conversion8/1 -> [I_PV], M_Ipv/1, Phase C/1

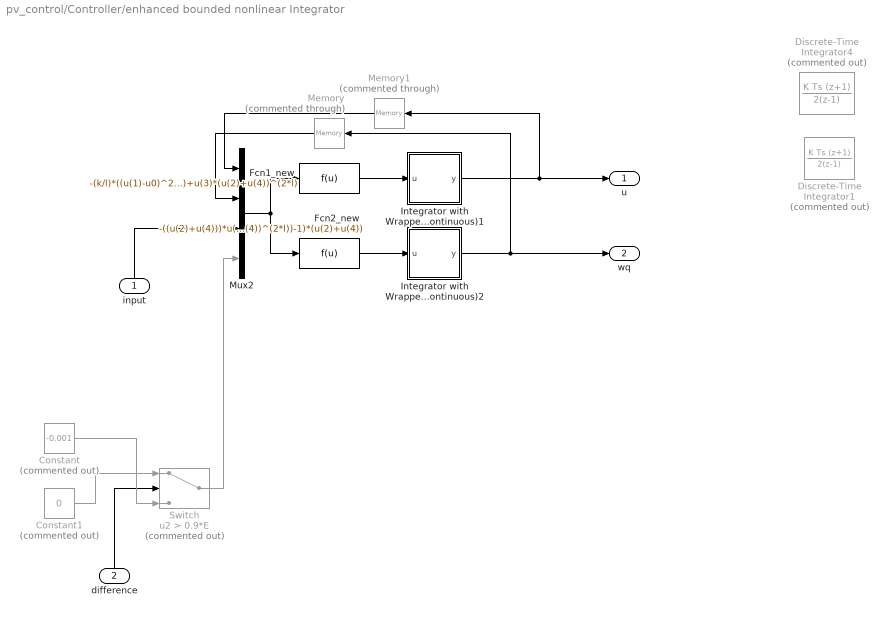
== system pv_control/Controller/enhanced bounded nonlinear Integrator ==
  input : Inport
  difference : Inport  Port=2
  Constant : Constant  Commented=on  Value=-0.001
  Constant1 : Constant  Commented=on  Value=0
  Discrete-Time Integrator1 : DiscreteIntegrator  Commented=on  IntegratorMethod=Integration: Trapezoidal  InitialCondition=1  SampleTime=Ts  ICPrevOutput=DiscIntNeverNeededParam  ICPrevScaledInput=DiscIntNeverNeededParam
  Discrete-Time Integrator4 : DiscreteIntegrator  Commented=on  IntegratorMethod=Integration: Trapezoidal  SampleTime=Ts  ICPrevOutput=DiscIntNeverNeededParam  ICPrevScaledInput=DiscIntNeverNeededParam
  "Fcn1_new " : Fcn  Expr=-(k/l)*((u(1)-u0)^2/(Vm)^2+(u(2)+u(4))^(2*l)-1)*(u(1)-u0)+u(3)*(u(2)+u(4))^(2*l)
  "Fcn2_new " : Fcn  Expr=-((u(2)+u(4)))*u(3)*(u(1)-u0)/(l*(Vm^2))-(k/l)*((u(1)-u0)^2/(Vm)^2+((u(2)+u(4))^(2*l))-1)*(u(2)+u(4))
  Integrator with Wrapped State (Discrete or Continuous)1 : Subsystem  AncestorBlock=|  LoadFcn=|  Variant=on  VariantControlMode=label  LabelModeActiveChoice=Discrete  mask(Integrator with Wrapped State (Discrete or Continuous)){WrappedStateUpperValue=2*Emax, WrappedStateLowerValue=-2*Emax, x0=0, Ts=Ts}
      AncestorBlock=|
      | peGeneralControl/Integrator with
      | Wrapped State
      | (Discrete or Continuous)
      LoadFcn=|
      | pe_sli_rtmsupport( 'loadfcn', gcbh );
      | pe.mask.callbackLoadFcn(gcbh);
      mask prompts: WrappedStateUpperValue "Wrapped state upper value:"; WrappedStateLowerValue "Wrapped state lower value:"; x0 "Initial condition:"; Ts "Sample time (-1 for inherited):"
      mask help:
      | This block models a discrete-time or continous-time integrator with a wrapped state.
      |
      | For inherited discrete-time, set Sample time to -1. For discrete-time, set Sample time to a positive value. For continuous-time, set Sample time to zero.
      |
      | Use this block to represent a Voltage Controlled Oscillator (VCO).
      mask init:
      | timeDomain = pe.mask.initializeIntegratorWrappedState(gcb,WrappedStateUpperValue,WrappedStateLowerValue,Ts);
      settings: CopyFcn=pe_sli_rtmsupport( 'copyfcn', gcbh );  DeleteFcn=pe_sli_rtmsupport( 'deletefcn', gcbh );  ModelCloseFcn=pe_sli_rtmsupport( 'modelclosefcn', gcbh );  PostSaveFcn=pe_sli_rtmsupport( 'postsavefcn', gcbh );  PreCopyFcn=pe_sli_rtmsupport( 'precopyfcn', gcbh );  OpenFcn=pe_sli_rtmsupport( 'openfcn', gcbh );  CloseFcn=pe_sli_rtmsupport( 'closefcn', gcbh );  PreDeleteFcn=pe_sli_rtmsupport( 'predeletefcn', gcbh );
      mask Help: web(nesl_help(gcbh))
      mask Display: pe.mask.drawIntegratorWrappedState;
  Integrator with Wrapped State (Discrete or Continuous)2 : Subsystem  AncestorBlock=|  LoadFcn=|  Variant=on  VariantControlMode=label  LabelModeActiveChoice=Discrete  mask(Integrator with Wrapped State (Discrete or Continuous)){WrappedStateUpperValue=2, WrappedStateLowerValue=-2, x0=1, Ts=Ts}
      AncestorBlock=|
      | peGeneralControl/Integrator with
      | Wrapped State
      | (Discrete or Continuous)
      LoadFcn=|
      | pe_sli_rtmsupport( 'loadfcn', gcbh );
      | pe.mask.callbackLoadFcn(gcbh);
      mask prompts: WrappedStateUpperValue "Wrapped state upper value:"; WrappedStateLowerValue "Wrapped state lower value:"; x0 "Initial condition:"; Ts "Sample time (-1 for inherited):"
      mask help:
      | This block models a discrete-time or continous-time integrator with a wrapped state.
      |
      | For inherited discrete-time, set Sample time to -1. For discrete-time, set Sample time to a positive value. For continuous-time, set Sample time to zero.
      |
      | Use this block to represent a Voltage Controlled Oscillator (VCO).
      mask init:
      | timeDomain = pe.mask.initializeIntegratorWrappedState(gcb,WrappedStateUpperValue,WrappedStateLowerValue,Ts);
      settings: CopyFcn=pe_sli_rtmsupport( 'copyfcn', gcbh );  DeleteFcn=pe_sli_rtmsupport( 'deletefcn', gcbh );  ModelCloseFcn=pe_sli_rtmsupport( 'modelclosefcn', gcbh );  PostSaveFcn=pe_sli_rtmsupport( 'postsavefcn', gcbh );  PreCopyFcn=pe_sli_rtmsupport( 'precopyfcn', gcbh );  OpenFcn=pe_sli_rtmsupport( 'openfcn', gcbh );  CloseFcn=pe_sli_rtmsupport( 'closefcn', gcbh );  PreDeleteFcn=pe_sli_rtmsupport( 'predeletefcn', gcbh );
      mask Help: web(nesl_help(gcbh))
      mask Display: pe.mask.drawIntegratorWrappedState;
  Memory : Memory  Commented=through  InitialCondition=1  LinearizeAsDelay=on
  Memory1 : Memory  Commented=through  LinearizeAsDelay=on
  Mux2 : Mux
  Switch : Switch  Commented=on  Criteria=u2 > Threshold  Threshold=0.9*E  SaturateOnIntegerOverflow=off  InputSameDT=off
  u : Outport
  wq : Outport  Port=2
  wires:
  input/1 -> Mux2/3
  Mux2/1 -> "Fcn2_new "/1, "Fcn1_new "/1
  difference/1 -> Switch/2
  "Fcn1_new "/1 -> Integrator with Wrapped State (Discrete or Continuous)1/1(u)
  "Fcn2_new "/1 -> Integrator with Wrapped State (Discrete or Continuous)2/1(u)
  Constant1/1 -> Switch/1
  Constant/1 -> Switch/3
  Integrator with Wrapped State (Discrete or Continuous)1/1(y) -> Memory1/1, u/1
  Integrator with Wrapped State (Discrete or Continuous)2/1(y) -> Memory/1, wq/1
  Memory1/1 -> Mux2/1
  Memory/1 -> Mux2/2
  Switch/1 -> Mux2/4

== system pv_control/DQ0 Transformation & P-w Droop/F to Oscilloscope ==
  In1 : Inport
  Calibrator5 : Subsystem
  Data Type Conversion3 : DataTypeConversion  OutDataTypeStr=double  SaturateOnIntegerOverflow=off  RndMeth=Floor
  Fcn1 : Fcn  Expr=u(1)*100
  Gain : Gain  Gain=1/(2*pi)
  Saturation4 : Saturate  UpperLimit=1  LowerLimit=0  OutDataTypeStr=double
  wires:
  In1/1 -> Gain/1
  Data Type Conversion3/1 -> ?
  Fcn1/1 -> Data Type Conversion3/1
  Saturation4/1 -> Fcn1/1
  Gain/1 -> Calibrator5/1(In1)
  Calibrator5/1(Out1) -> Saturation4/1

== system pv_control/DQ0 Transformation & P-w Droop/P to oscilloscope ==
  In1 : Inport
  Calibrator1 : Subsystem
  Data Type Conversion1 : DataTypeConversion  OutDataTypeStr=double  SaturateOnIntegerOverflow=off  RndMeth=Floor
  Fcn3 : Fcn  Expr=u(1)*100
  Saturation1 : Saturate  UpperLimit=1  LowerLimit=0  OutDataTypeStr=double
  wires:
  Fcn3/1 -> Data Type Conversion1/1
  Calibrator1/1(Out1) -> Saturation1/1
  In1/1 -> Calibrator1/1(In1)
  Saturation1/1 -> Fcn3/1
  Data Type Conversion1/1 -> ?

== system pv_control/DQ0 Transformation & P-w Droop/Q to oscilloscope ==
  In1 : Inport
  Calibrator2 : Subsystem
  Data Type Conversion1 : DataTypeConversion  OutDataTypeStr=double  SaturateOnIntegerOverflow=off  RndMeth=Floor
  Fcn3 : Fcn  Expr=u(1)*100
  Saturation1 : Saturate  UpperLimit=1  LowerLimit=0  OutDataTypeStr=double
  wires:
  Saturation1/1 -> Fcn3/1
  Fcn3/1 -> Data Type Conversion1/1
  In1/1 -> Calibrator2/1(In1)
  Calibrator2/1(Out1) -> Saturation1/1
  Data Type Conversion1/1 -> ?

== system pv_control/DQ0 Transformation & P-w Droop/Vrms to oscilloscope ==
  In1 : Inport
  0-1 regulator for Vrms : Subsystem
  Data Type Conversion2 : DataTypeConversion  OutDataTypeStr=double  SaturateOnIntegerOverflow=off  RndMeth=Floor
  Fcn4 : Fcn  Expr=u(1)*100
  Saturation2 : Saturate  UpperLimit=1  LowerLimit=0  OutDataTypeStr=double
  wires:
  Data Type Conversion2/1 -> ?
  Saturation2/1 -> Fcn4/1
  Fcn4/1 -> Data Type Conversion2/1
  0-1 regulator for Vrms/1(Out1) -> Saturation2/1
  In1/1 -> 0-1 regulator for Vrms/1(In1)

== system pv_control/Controller/enhanced bounded nonlinear Integrator/Integrator with Wrapped State (Discrete or Continuous)1 ==
  u : Inport
  Continuous : Subsystem  VariantControl=Continuous
  Discrete : Subsystem  VariantControl=Discrete
  y : Outport

== system pv_control/Controller/enhanced bounded nonlinear Integrator/Integrator with Wrapped State (Discrete or Continuous)2 ==
  u : Inport
  Continuous : Subsystem  VariantControl=Continuous
  Discrete : Subsystem  VariantControl=Discrete
  y : Outport

== system pv_control/DQ0 Transformation & P-w Droop/F to Oscilloscope/Calibrator5 ==
  In1 : Inport
  Add : Sum
  Fcn1 : Fcn  Expr=u(1)
  Fcn2 : Fcn  Expr=0.5*u(1)
  Offset_ia : Constant  Value=-49
  Out1 : Outport
  wires:
  In1/1 -> Fcn1/1
  Offset_ia/1 -> Add/2
  Fcn1/1 -> Add/1
  Add/1 -> Fcn2/1
  Fcn2/1 -> Out1/1

== system pv_control/DQ0 Transformation & P-w Droop/P to oscilloscope/Calibrator1 ==
  In1 : Inport
  Add : Sum
  Fcn1 : Fcn  Expr=u(1)
  Fcn2 : Fcn  Expr=(1/40)*u(1)
  Offset_ia : Constant  Value=0
  Out1 : Outport
  wires:
  Fcn2/1 -> Out1/1
  Add/1 -> Fcn2/1
  Fcn1/1 -> Add/1
  Offset_ia/1 -> Add/2
  In1/1 -> Fcn1/1

== system pv_control/DQ0 Transformation & P-w Droop/Q to oscilloscope/Calibrator2 ==
  In1 : Inport
  Add : Sum
  Fcn1 : Fcn  Expr=-u(1)
  Fcn2 : Fcn  Expr=(1/2.3)*u(1)
  Offset_ia : Constant  Value=0
  Out1 : Outport
  wires:
  Fcn2/1 -> Out1/1
  Add/1 -> Fcn2/1
  Fcn1/1 -> Add/1
  Offset_ia/1 -> Add/2
  In1/1 -> Fcn1/1

== system pv_control/DQ0 Transformation & P-w Droop/Vrms to oscilloscope/0-1 regulator for Vrms ==
  In1 : Inport
  Add : Sum
  Fcn1 : Fcn  Expr=u(1)
  Fcn2 : Fcn  Expr=(1/10.6)*u(1)
  Offset_ia : Constant  Value=0
  Out1 : Outport
  wires:
  In1/1 -> Fcn1/1
  Offset_ia/1 -> Add/2
  Fcn1/1 -> Add/1
  Add/1 -> Fcn2/1
  Fcn2/1 -> Out1/1

== system pv_control/Controller/enhanced bounded nonlinear Integrator/Integrator with Wrapped State (Discrete or Continuous)1/Continuous ==
  u : Inport
  Integrator : Integrator  InitialCondition=x0  WrapState=on  WrappedStateUpperValue=WrappedStateUpperValue  WrappedStateLowerValue=WrappedStateLowerValue
  y : Outport
  wires:
  Integrator/1 -> y/1
  u/1 -> Integrator/1

== system pv_control/Controller/enhanced bounded nonlinear Integrator/Integrator with Wrapped State (Discrete or Continuous)1/Discrete ==
  u : Inport
  Integrator : DiscreteIntegrator  InitialCondition=x0  SampleTime=Ts  ICPrevOutput=DiscIntNeverNeededParam  ICPrevScaledInput=DiscIntNeverNeededParam
  y : Outport
  wires:
  Integrator/1 -> y/1
  u/1 -> Integrator/1

== system pv_control/Controller/enhanced bounded nonlinear Integrator/Integrator with Wrapped State (Discrete or Continuous)2/Continuous ==
  u : Inport
  Integrator : Integrator  InitialCondition=x0  WrapState=on  WrappedStateUpperValue=WrappedStateUpperValue  WrappedStateLowerValue=WrappedStateLowerValue
  y : Outport
  wires:
  u/1 -> Integrator/1
  Integrator/1 -> y/1

== system pv_control/Controller/enhanced bounded nonlinear Integrator/Integrator with Wrapped State (Discrete or Continuous)2/Discrete ==
  u : Inport
  Integrator : DiscreteIntegrator  InitialCondition=x0  SampleTime=Ts  ICPrevOutput=DiscIntNeverNeededParam  ICPrevScaledInput=DiscIntNeverNeededParam
  y : Outport
  wires:
  u/1 -> Integrator/1
  Integrator/1 -> y/1
